simulink model "origin"  (R2021b)
settings: Solver=VariableStepAuto  StartTime=0.0  StopTime=10.0  FixedStep=0.0001  RelTol=1e-3
settings Model: PauseTimes=0.1  Creator=O  LastModifiedBy=ojiken

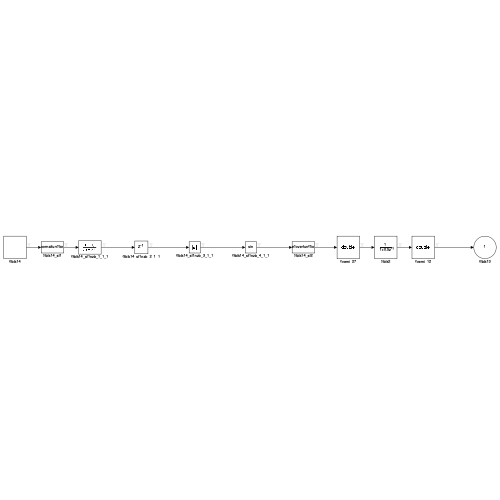
[thumbnail: Simulink's stored preview of the top-level diagram]
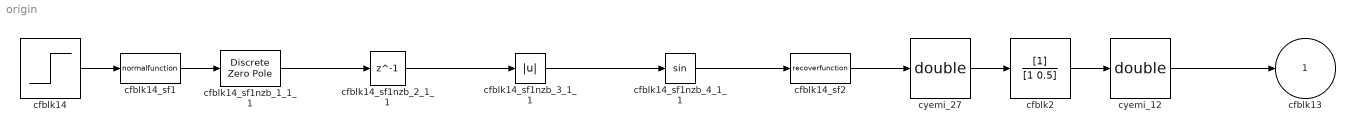
== system origin ==
  cfblk14 : Step  Time=[6.000000]  Before=[769690289.111915]  After=[-653636333.758309]  SampleTime=0
  cfblk14_sf1 : S-Function  FunctionName=normalfunction  SFunctionDeploymentMode=off  EnableBusSupport=off
  cfblk14_sf1nzb_1_1_1 : DiscreteZeroPole  Poles=[0 0.5]  Gain=1  SampleTime=-1
  cfblk14_sf1nzb_2_1_1 : Delay  DelayLength=1  InitialCondition=0
  cfblk14_sf1nzb_3_1_1 : Abs
  cfblk14_sf1nzb_4_1_1 : Trigonometry
  cfblk14_sf2 : S-Function  FunctionName=recoverfunction  SFunctionDeploymentMode=off  EnableBusSupport=off
  cfblk2 : DiscreteFilter  SampleTime=1
  cyemi_12 : DataTypeConversion  OutDataTypeStr=double
  cyemi_27 : DataTypeConversion  OutDataTypeStr=double
  cfblk13 : Outport
  wires:
  cfblk2/1 -> cyemi_12/1
  cfblk14_sf1nzb_2_1_1/1 -> cfblk14_sf1nzb_3_1_1/1
  cfblk14_sf1nzb_3_1_1/1 -> cfblk14_sf1nzb_4_1_1/1
  cyemi_12/1 -> cfblk13/1
  cyemi_27/1 -> cfblk2/1
  cfblk14_sf1nzb_1_1_1/1 -> cfblk14_sf1nzb_2_1_1/1
  cfblk14/1 -> cfblk14_sf1/1
  cfblk14_sf1/1 -> cfblk14_sf1nzb_1_1_1/1
  cfblk14_sf1nzb_4_1_1/1 -> cfblk14_sf2/1
  cfblk14_sf2/1 -> cyemi_27/1
